simulink model "fdatool9"  (Simulink 5.1)
settings: Solver=ode45  StartTime=0.0  StopTime=10.0  RelTol=1e-3
libraries: dspsigops x8
settings Model: Creator=svenhoffmann  LastModifiedBy=svenhoffmann  ExtModeAutoUpdateStatusClock=off  BooleanDataType=on  ProdHWDeviceType=Microprocessor

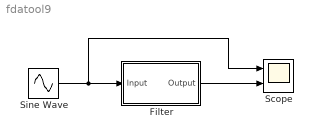
== system fdatool9 ==
  Filter : Subsystem  Tag=FilterWizardSubSystem
  Scope : Scope  NumInputPorts=2
      settings: YMin=-5~-5  YMax=5~5
  Sine Wave : Sin  Amplitude=100  Frequency=2*pi*210  SampleTime=1/1000
  wires:
  Sine Wave/1 -> Scope/1, Filter/1(Input)
  Filter/1(Output) -> Scope/2

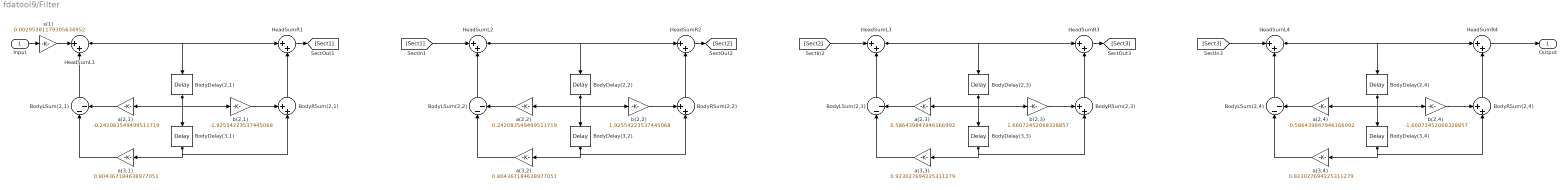
== system fdatool9/Filter ==
  Input : Inport
  BodyDelay(2,1) : dspsigops/Delay  Orientation=down  dly_unit=Samples  delay=1  ic_detail=off  dif_ic_for_ch=off  dif_ic_for_dly=off  ic=0  reset_popup=None
  BodyDelay(2,2) : dspsigops/Delay  Orientation=down  dly_unit=Samples  delay=1  ic_detail=off  dif_ic_for_ch=off  dif_ic_for_dly=off  ic=0  reset_popup=None
  BodyDelay(2,3) : dspsigops/Delay  Orientation=down  dly_unit=Samples  delay=1  ic_detail=off  dif_ic_for_ch=off  dif_ic_for_dly=off  ic=0  reset_popup=None
  BodyDelay(2,4) : dspsigops/Delay  Orientation=down  dly_unit=Samples  delay=1  ic_detail=off  dif_ic_for_ch=off  dif_ic_for_dly=off  ic=0  reset_popup=None
  BodyDelay(3,1) : dspsigops/Delay  Orientation=down  dly_unit=Samples  delay=1  ic_detail=off  dif_ic_for_ch=off  dif_ic_for_dly=off  ic=0  reset_popup=None
  BodyDelay(3,2) : dspsigops/Delay  Orientation=down  dly_unit=Samples  delay=1  ic_detail=off  dif_ic_for_ch=off  dif_ic_for_dly=off  ic=0  reset_popup=None
  BodyDelay(3,3) : dspsigops/Delay  Orientation=down  dly_unit=Samples  delay=1  ic_detail=off  dif_ic_for_ch=off  dif_ic_for_dly=off  ic=0  reset_popup=None
  BodyDelay(3,4) : dspsigops/Delay  Orientation=down  dly_unit=Samples  delay=1  ic_detail=off  dif_ic_for_ch=off  dif_ic_for_dly=off  ic=0  reset_popup=None
  BodyLSum(2,1) : Sum  Orientation=up  Inputs=|--  SaturateOnIntegerOverflow=on  InputSameDT=on
  BodyLSum(2,2) : Sum  Orientation=up  Inputs=|--  SaturateOnIntegerOverflow=on  InputSameDT=on
  BodyLSum(2,3) : Sum  Orientation=up  Inputs=|--  SaturateOnIntegerOverflow=on  InputSameDT=on
  BodyLSum(2,4) : Sum  Orientation=up  Inputs=|--  SaturateOnIntegerOverflow=on  InputSameDT=on
  BodyRSum(2,1) : Sum  Orientation=up  Inputs=++|  SaturateOnIntegerOverflow=on  InputSameDT=on
  BodyRSum(2,2) : Sum  Orientation=up  Inputs=++|  SaturateOnIntegerOverflow=on  InputSameDT=on
  BodyRSum(2,3) : Sum  Orientation=up  Inputs=++|  SaturateOnIntegerOverflow=on  InputSameDT=on
  BodyRSum(2,4) : Sum  Orientation=up  Inputs=++|  SaturateOnIntegerOverflow=on  InputSameDT=on
  HeadSumL{1..4} (4 alike) : Sum  Inputs=|++  SaturateOnIntegerOverflow=on  InputSameDT=on
  HeadSumR{1..4} (4 alike) : Sum  Inputs=|++  SaturateOnIntegerOverflow=on  InputSameDT=on
  a(2,1) : Gain  Orientation=left  Gain=-0.242083549499511719  SaturateOnIntegerOverflow=on
  a(2,2) : Gain  Orientation=left  Gain=0.242083549499511719  SaturateOnIntegerOverflow=on
  a(2,3) : Gain  Orientation=left  Gain=0.586439847946166992  SaturateOnIntegerOverflow=on
  a(2,4) : Gain  Orientation=left  Gain=-0.586439847946166992  SaturateOnIntegerOverflow=on
  a(3,1) : Gain  Orientation=left  Gain=0.804367184638977051  SaturateOnIntegerOverflow=on
  a(3,2) : Gain  Orientation=left  Gain=0.804367184638977051  SaturateOnIntegerOverflow=on
  a(3,3) : Gain  Orientation=left  Gain=0.923027694225311279  SaturateOnIntegerOverflow=on
  a(3,4) : Gain  Orientation=left  Gain=0.923027694225311279  SaturateOnIntegerOverflow=on
  b(2,1) : Gain  Gain=-1.92554223537445068  SaturateOnIntegerOverflow=on
  b(2,2) : Gain  Gain=1.92554223537445068  SaturateOnIntegerOverflow=on
  b(2,3) : Gain  Gain=1.66072452068328857  SaturateOnIntegerOverflow=on
  b(2,4) : Gain  Gain=-1.66072452068328857  SaturateOnIntegerOverflow=on
  s(1) : Gain  Gain=0.00295381179305634952  SaturateOnIntegerOverflow=on
  Output : Outport
  wires:
  Input/1 -> s(1)/1
  s(1)/1 -> HeadSumL1/1
  HeadSumL1/1 -> BodyDelay(2,1)/1, HeadSumR1/1
  HeadSumR1/1 -> [Sect1]
  BodyDelay(2,1)/1 -> a(2,1)/1, b(2,1)/1, BodyDelay(3,1)/1
  a(2,1)/1 -> BodyLSum(2,1)/2
  b(2,1)/1 -> BodyRSum(2,1)/1
  BodyLSum(2,1)/1 -> HeadSumL1/2
  BodyRSum(2,1)/1 -> HeadSumR1/2
  BodyDelay(3,1)/1 -> a(3,1)/1, BodyRSum(2,1)/2
  a(3,1)/1 -> BodyLSum(2,1)/1
  [Sect1] -> HeadSumL2/1
  HeadSumL2/1 -> BodyDelay(2,2)/1, HeadSumR2/1
  HeadSumR2/1 -> [Sect2]
  BodyDelay(2,2)/1 -> a(2,2)/1, b(2,2)/1, BodyDelay(3,2)/1
  a(2,2)/1 -> BodyLSum(2,2)/2
  b(2,2)/1 -> BodyRSum(2,2)/1
  BodyLSum(2,2)/1 -> HeadSumL2/2
  BodyRSum(2,2)/1 -> HeadSumR2/2
  BodyDelay(3,2)/1 -> a(3,2)/1, BodyRSum(2,2)/2
  a(3,2)/1 -> BodyLSum(2,2)/1
  [Sect2] -> HeadSumL3/1
  HeadSumL3/1 -> BodyDelay(2,3)/1, HeadSumR3/1
  HeadSumR3/1 -> [Sect3]
  BodyDelay(2,3)/1 -> a(2,3)/1, b(2,3)/1, BodyDelay(3,3)/1
  a(2,3)/1 -> BodyLSum(2,3)/2
  b(2,3)/1 -> BodyRSum(2,3)/1
  BodyLSum(2,3)/1 -> HeadSumL3/2
  BodyRSum(2,3)/1 -> HeadSumR3/2
  BodyDelay(3,3)/1 -> a(3,3)/1, BodyRSum(2,3)/2
  a(3,3)/1 -> BodyLSum(2,3)/1
  [Sect3] -> HeadSumL4/1
  HeadSumL4/1 -> BodyDelay(2,4)/1, HeadSumR4/1
  HeadSumR4/1 -> Output/1
  BodyDelay(2,4)/1 -> a(2,4)/1, b(2,4)/1, BodyDelay(3,4)/1
  a(2,4)/1 -> BodyLSum(2,4)/2
  b(2,4)/1 -> BodyRSum(2,4)/1
  BodyLSum(2,4)/1 -> HeadSumL4/2
  BodyRSum(2,4)/1 -> HeadSumR4/2
  BodyDelay(3,4)/1 -> a(3,4)/1, BodyRSum(2,4)/2
  a(3,4)/1 -> BodyLSum(2,4)/1
